simulink model "db4_14"  (R2018a)
settings: Solver=ode45  StartTime=0.0  StopTime=8  MaxStep=3e-5  RelTol=1e-3  AbsTol=1e-3
values from neighbouring files (symbols this model uses):
  Tc = str2num(get(findobj('Tag','variable6'),'String'))    [graficas_a.m]    (also in simulaciones.m = str2num(get(findobj('Tag','variable5'),'String')))
  Wref = str2num(get(findobj('Tag','variable5'),'String'))    [graficas_a.m]    (also in simulaciones.m)
libraries: simulink x2
settings Model: ExtModeTrigMode=oneshot  ExtModeArmWhenConnect=off  Creator=Lac User  LastModifiedBy=Matias
settings SolverCC: AutoScaleAbsTol=off
settings DataIOCC: SaveFormat=Array  SignalLoggingSaveFormat=ModelDataLogs  SaveOutput=off  SaveTime=off
settings OptimizationCC: BlockReduction=off  BooleanDataType=off  LifeSpan=inf
settings DebuggingCC: SaveWithParameterizedLinksMsg=none  UnderspecifiedInitializationDetection=Classic  MergeDetectMultiDrivingBlocksExec=none  SignalResolutionControl=TryResolveAllWithWarning  MultiTaskDSMMsg=warning  MultiTaskCondExecSysMsg=none  SFUnexpectedBacktrackingDiag=warning  SFNoUnconditionalDefaultTransitionDiag=warning  SFExecutionAtInitializationDiag=none
settings HardwareCC: ProdBitPerPointer=32  ProdBitPerSizeT=32  ProdBitPerPtrDiffT=32  ProdLargestAtomicFloat=None  ProdIntDivRoundTo=Undefined  ProdEndianess=Unspecified  ProdWordSize=32  ProdHWDeviceType=32-bit Generic  TargetUnknown=on
settings ModelReferenceCC: PropagateSignalLabelsOutOfModel=off
settings RTWCC: TemplateMakefile=grt_vc.tmf
settings CodeAppCC: StateflowObjectComments=on
settings GRTTargetCC: TargetLangStandard=C89/C90 (ANSI)  GeneratePreprocessorConditionals=Disable all  CombineOutputUpdateFcns=off  GRTInterface=on
settings ConfigComp: CovMetricSettings=dw  CovHtmlReporting=on  CovSaveCumulativeToWorkspaceVar=on  CovSaveSingleToWorkspaceVar=on  CovExternalEMLEnable=off

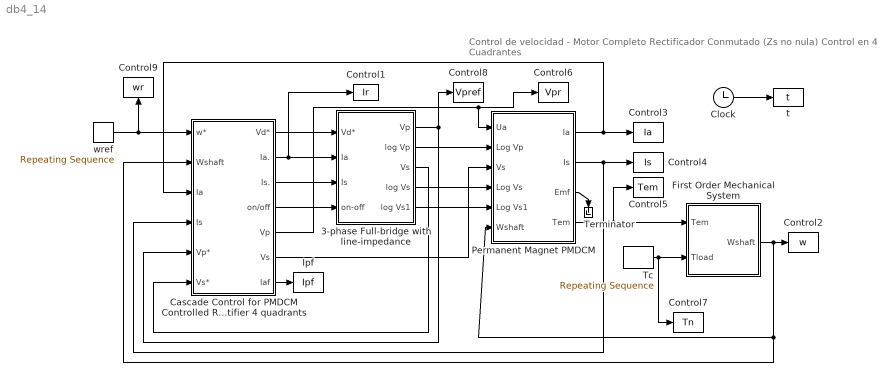
== system db4_14 ==
  note: Control de velocidad - Motor Completo
      | Rectificador Conmutado (Zs no nula) Control en 4 Cuadrantes
  3-phase Full-bridge with line-impedance : Subsystem  mask(3-phase Full-bridge with line-impedance){Vph=220, f=50, Rd=0.05, Ld=0.003, Rs=6e-05, Ls=2e-05}
      mask prompts: Vph "RMS Phase Voltage [V]:"; f "Frecuency [Hz]:"; Rd "Armature Resistance [Ohms]:"; Ld "Armature Inductance  [Hy]:"; Rs "Line Resistance [Ohms]:"; Ls "Line Inductance [Hy]:"
  "Cascade Control for PMDCM Controlled Rectifier 4 quadrants " : Subsystem  mask(Cascade Control (Speed and Current) for PMDCM Controlled Rectifier four quadrants){Kpn=283.88, TIn=0.3135, Kpi=0.08, TIi=0.027, Ktn=0.06, Tfn=0.008, Kti=1, Tfi=0.008, k=6.7851, Ian=319.6936}
      mask prompts: Kpn "Speed Proportional Gain:"; TIn "Speed Integral Gain:"; Kpi "Current Proportional Gain:"; TIi "Current Integral Gain:"; Ktn "Speed-sensor Proportional Gain:"; Tfn "Speed-sensor Integral Gain:"; Kti "Current-sensor Proportional Gain:"; Tfi "Current-sensor Integral Gain:"; k "Motor Constant:"; Ian "Rated Armature Current [Amp]:"
  Clock : Clock
  Control1 : ToWorkspace  VariableName=Ir
      settings: MaxDataPoints=300000
  Control2 : ToWorkspace  VariableName=w
      settings: MaxDataPoints=300000
  Control3 : ToWorkspace  VariableName=Ia
      settings: MaxDataPoints=300000
  Control4 : ToWorkspace  VariableName=Is
      settings: MaxDataPoints=300000
  Control5 : ToWorkspace  VariableName=Tem
      settings: MaxDataPoints=300000
  Control6 : ToWorkspace  VariableName=Vpr
      settings: MaxDataPoints=300000
  Control7 : ToWorkspace  VariableName=Tn
      settings: MaxDataPoints=300000
  Control8 : ToWorkspace  VariableName=Vpref
      settings: MaxDataPoints=300000
  Control9 : ToWorkspace  VariableName=wr
      settings: MaxDataPoints=300000
  First Order Mechanical System : Subsystem  mask(First Order Mechanical System){J=15, b=1.1, wor=0}
      mask prompts: J "Inertia [Kgm]:"; b "Friction Coeficient [Nm seg/rad]:"; wor "Speed Initial Condition [rad/sec]:"
      mask help:
      | This block solves the following differential equation:
      |
      | dW(t)/dt = - W(t)/J + (Tm -- bW(t) -- Load )/J
      | W(0)=W0
  Ipf : ToWorkspace  VariableName=Ipf
      settings: MaxDataPoints=300000
  Permanent Magnet PMDCM : Subsystem  mask(Permanent Magnet PMDCM){La=0.003, Ra=0.05, k=6.7851, ic=0, Ls=2e-05, Rs=6e-05}
      mask prompts: La "Armature Inductance  [Hy]:"; Ra "Armature Resistance [Ohms]:"; k "Motor Constant:"; ic "Armature Current Initial Condition [Amp]:"; Ls "Line Inductance [Hy]:"; Rs "Line Resistance [Ohms]:"
  Tc : simulink/Sources/Repeating Sequence  rep_seq_t=[0 7.5 7.9 8 9 9.1 10 13.5 14]  rep_seq_y="[0 0    0 -Tc -Tc -Tc -Tc -Tc 0]"
  Terminator : Terminator
  t : ToWorkspace  VariableName=t
      settings: MaxDataPoints=300000
  wref : simulink/Sources/Repeating Sequence  rep_seq_t="[0     1.5  2.5  3 4.5   5    6     8    9    10 11   12 15]"  rep_seq_y="[Wref Wref Wref  0  0    0   Wref   Wref Wref Wref  Wref   -Wref -Wref]"
  wires:
  wref/1 -> Control9/1, "Cascade Control for PMDCM Controlled Rectifier 4 quadrants "/1(w*)
  "Cascade Control for PMDCM Controlled Rectifier 4 quadrants "/7(Iaf) -> Ipf/1
  First Order Mechanical System/1(Wshaft) -> Permanent Magnet PMDCM/6(Wshaft), "Cascade Control for PMDCM Controlled Rectifier 4 quadrants "/2(Wshaft), Control2/1
  "Cascade Control for PMDCM Controlled Rectifier 4 quadrants "/1(Vd*) -> 3-phase Full-bridge with line-impedance/1(Vd*)
  "Cascade Control for PMDCM Controlled Rectifier 4 quadrants "/4(on/off) -> 3-phase Full-bridge with line-impedance/4(on-off)
  "Cascade Control for PMDCM Controlled Rectifier 4 quadrants "/3(Is.) -> 3-phase Full-bridge with line-impedance/3(Is)
  3-phase Full-bridge with line-impedance/3(Vs) -> "Cascade Control for PMDCM Controlled Rectifier 4 quadrants "/6(Vs*)
  "Cascade Control for PMDCM Controlled Rectifier 4 quadrants "/6(Vs) -> Permanent Magnet PMDCM/3(Vs)
  3-phase Full-bridge with line-impedance/5(log Vs1) -> Permanent Magnet PMDCM/5(Log Vs1)
  3-phase Full-bridge with line-impedance/4(log Vs) -> Permanent Magnet PMDCM/4(Log Vs)
  "Cascade Control for PMDCM Controlled Rectifier 4 quadrants "/5(Vp) -> Permanent Magnet PMDCM/1(Ua), Control6/1
  3-phase Full-bridge with line-impedance/2(log Vp) -> Permanent Magnet PMDCM/2(Log Vp)
  "Cascade Control for PMDCM Controlled Rectifier 4 quadrants "/2(Ia.) -> 3-phase Full-bridge with line-impedance/2(Ia), Control1/1
  3-phase Full-bridge with line-impedance/1(Vp) -> "Cascade Control for PMDCM Controlled Rectifier 4 quadrants "/5(Vp*), Control8/1
  Permanent Magnet PMDCM/3(Emf) -> Terminator/1
  Permanent Magnet PMDCM/2(Is) -> Control4/1, "Cascade Control for PMDCM Controlled Rectifier 4 quadrants "/4(Is)
  Permanent Magnet PMDCM/1(Ia) -> Control3/1, "Cascade Control for PMDCM Controlled Rectifier 4 quadrants "/3(Ia)
  Permanent Magnet PMDCM/4(Tem) -> First Order Mechanical System/1(Tem), Control5/1
  Tc/1 -> First Order Mechanical System/2(Tload), Control7/1
  Clock/1 -> t/1

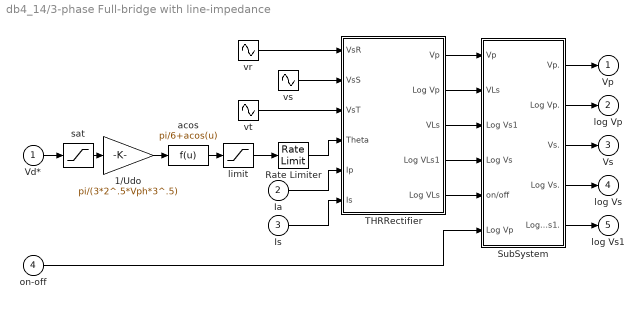
== system db4_14/3-phase Full-bridge with line-impedance ==
  Vd* : Inport
  Ia : Inport  Port=2
  Is : Inport  Port=3
  on-off : Inport  Port=4
  1/Udo : Gain  Gain=pi/(3*2^.5*Vph*3^.5)  SaturateOnIntegerOverflow=on  OutDataTypeStr=Inherit: Same as input  ParamDataTypeStr=Inherit: Same as input
  Rate Limiter : RateLimiter  RisingSlewLimit=8000  FallingSlewLimit=-8000
  SubSystem : Subsystem
  THRRectifier : Subsystem
      mask Display:
      | plot([0.3 0.7 0.5 0.3],[0.4 0.4 0.6 0.4])
      | plot([0.3 0.7 ],[0.6 0.6])
      | plot([0.5 0.5 ],[0.6 0.7])
      | plot([0.5 0.5 ],[0.3 0.4])
      | plot([0.35 0.5],[0.7 0.6])
      | plot([0.25 0.35 ],[0.7 0.7])
  acos : Fcn  Expr=pi/6+acos(u)
  limit : Saturate  UpperLimit=pi*6.999/6  LowerLimit=pi/5.998
  sat : Saturate  UpperLimit=(3*2^.5*3^.5*Vph)/pi  LowerLimit=-(3*2^.5*3^.5*Vph)/pi
  vr : Sin  Amplitude=Vph*(2^.5)  Frequency=2*f*pi  SampleTime=0
  vs : Sin  Amplitude=Vph*(2^.5)  Frequency=2*pi*f  Phase=-(2/3)*pi  SampleTime=0
  vt : Sin  Amplitude=Vph*(2^.5)  Frequency=2*pi*f  Phase=-(4/3)*pi  SampleTime=0
  Vp : Outport
  log Vp : Outport  Port=2
  Vs : Outport  Port=3
  log Vs : Outport  Port=4
  log Vs1 : Outport  Port=5
  wires:
  1/Udo/1 -> acos/1
  acos/1 -> limit/1
  vt/1 -> THRRectifier/3(VsT)
  vs/1 -> THRRectifier/2(VsS)
  vr/1 -> THRRectifier/1(VsR)
  Vd*/1 -> sat/1
  Ia/1 -> THRRectifier/5(Ip)
  Is/1 -> THRRectifier/6(Is)
  sat/1 -> 1/Udo/1
  limit/1 -> Rate Limiter/1
  THRRectifier/1(Vp) -> SubSystem/1(Vp)
  THRRectifier/2(Log Vp) -> SubSystem/2(VLs)
  THRRectifier/3(VLs) -> SubSystem/3(Log Vs1)
  THRRectifier/4(Log VLs1) -> SubSystem/4(Log Vs)
  THRRectifier/5(Log VLs) -> SubSystem/5(on/off)
  on-off/1 -> SubSystem/6(Log Vp)
  SubSystem/2(Log Vp.) -> log Vp/1
  SubSystem/3(Vs.) -> Vs/1
  SubSystem/4(Log Vs.) -> log Vs/1
  SubSystem/5(Log Vs1.) -> log Vs1/1
  SubSystem/1(Vp.) -> Vp/1
  Rate Limiter/1 -> THRRectifier/4(Theta)

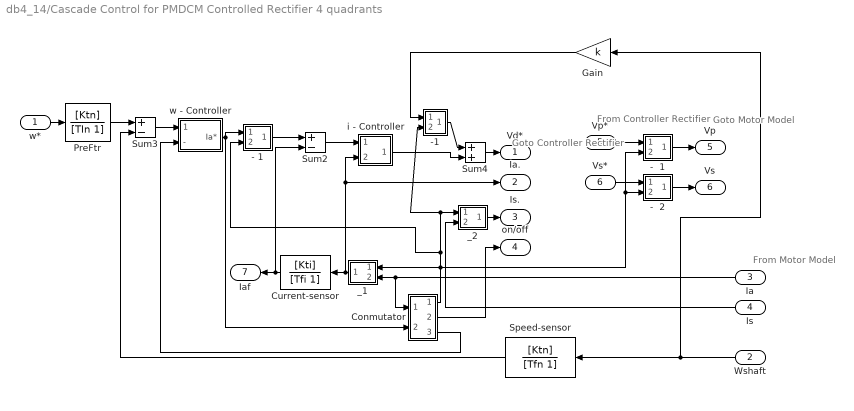
== system db4_14/Cascade Control for PMDCM Controlled Rectifier 4 quadrants  ==
  note: From Controller
      | Rectifier
  note: Goto Motor
      | Model
  note: Goto Controller
      | Rectifier
  note: From Motor
      | Model
  w* : Inport
  Wshaft : Inport  Port=2
  Ia : Inport  Port=3
  Is : Inport  Port=4
  Vp* : Inport  Port=5
  Vs* : Inport  Port=6
  -  1 : Subsystem
      mask Display: disp('-1')
  -  2 : Subsystem
      mask Display: disp('-1')
  - 1 : Subsystem
      mask Display: disp('-1')
  -1 : Subsystem
      mask Display: disp('-1')
  Conmutator : Subsystem
  Current-sensor : TransferFcn  Numerator=[Kti]  Denominator=[Tfi 1]
  Gain : Gain  Gain=k  SaturateOnIntegerOverflow=on  OutDataTypeStr=Inherit: Same as input  ParamDataTypeStr=Inherit: Same as input
  PreFtr : TransferFcn  Numerator=[Ktn]  Denominator=[TIn 1]
  Speed-sensor : TransferFcn  Numerator=[Ktn]  Denominator=[Tfn 1]
  Sum2 : Sum  Inputs=+-  SaturateOnIntegerOverflow=on  InputSameDT=on  OutDataTypeStr=Inherit: Same as first input
  Sum3 : Sum  Inputs=+-  SaturateOnIntegerOverflow=on  InputSameDT=on  OutDataTypeStr=Inherit: Same as first input
  Sum4 : Sum  SaturateOnIntegerOverflow=on  InputSameDT=on  OutDataTypeStr=Inherit: Same as first input
  _1 : Subsystem
      mask Display: disp('-1')
  _2 : Subsystem
      mask Display: disp('-1')
  i - Controller : Subsystem
      mask Display: plot([0 .01  5],[0 2 4])
  w - Controller : Subsystem
      mask Display:
      | plot([0.1 .1  0.6],[0.1 .5 .9])
      | plot([0.85 0.95],[0.65 0.65])
      | plot([0.8 0.85],[0.75 0.65])
      | plot([0.95 1],[0.65 0.75])
      | plot([0.85 0.95],[0.35 0.35])
      | plot([0.80 0.85],[0.25 0.35])
      | plot([0.95 1],[0.35 0.25])
      | plot([0.7 1], [0.5 .5])
      | plot([0 0], [0 1])
      | plot([0 0.7], [1 1])
      | plot([0.7 0.7], [0 1])
      | plot([0 0.7], [0 0])
  Vd* : Outport
  Ia. : Outport  Port=2
  Is. : Outport  Port=3
  on/off : Outport  Port=4
  Vp : Outport  Port=5
  Vs : Outport  Port=6
  Iaf : Outport  Port=7
  wires:
  Speed-sensor/1 -> Sum3/2
  PreFtr/1 -> Sum3/1
  _1/1(out_1) -> Current-sensor/1, i - Controller/2(Ia), Ia./1
  Sum2/1 -> i - Controller/1(Iaref - Iaf)
  Sum3/1 -> w - Controller/1(w - Iref)
  Conmutator/3(Ir = 0) -> w - Controller/2(-)
  w*/1 -> PreFtr/1
  - 1/1(out_1) -> Sum2/1
  Conmutator/2(Vp*1) -> on/off/1
  w - Controller/1(Ia*) -> - 1/1(in_1), Conmutator/2(Iaref)
  Conmutator/1(Vp*) -> - 1/2(in_2), _2/1(in_2), -1/2(in_2), -  2/2(in_2), -  1/2(in_2), _1/1(in_2)
  Vp*/1 -> -  1/1(in_1)
  Vs*/1 -> -  2/1(in_1)
  -  1/1(out_1) -> Vp/1
  -  2/1(out_1) -> Vs/1
  _2/1(out_1) -> Is./1
  Is/1 -> _2/2(in_1)
  Gain/1 -> -1/1(in_1)
  -1/1(out_1) -> Sum4/1
  i - Controller/1(Vp*) -> Sum4/2
  Sum4/1 -> Vd*/1
  Ia/1 -> _1/2(in_1), Conmutator/1(Ia)
  Wshaft/1 -> Speed-sensor/1, Gain/1
  Current-sensor/1 -> Sum2/2, Iaf/1

== system db4_14/First Order Mechanical System ==
  Tem : Inport
  Tload : Inport  Port=2
  Gain : Gain  Gain=1/J  SaturateOnIntegerOverflow=on  OutDataTypeStr=Inherit: Same as input  ParamDataTypeStr=Inherit: Same as input
  Gain1 : Gain  Gain=b  SaturateOnIntegerOverflow=on  OutDataTypeStr=Inherit: Same as input  ParamDataTypeStr=Inherit: Same as input
  Integrator : Integrator  InitialCondition=wor
  Sum : Sum  Inputs=+--  SaturateOnIntegerOverflow=on  InputSameDT=on  OutDataTypeStr=Inherit: Same as first input
  Wshaft : Outport
  wires:
  Integrator/1 -> Wshaft/1, Gain1/1
  Gain1/1 -> Sum/3
  Gain/1 -> Integrator/1
  Sum/1 -> Gain/1
  Tem/1 -> Sum/1
  Tload/1 -> Sum/2

== system db4_14/Permanent Magnet PMDCM ==
  Ua : Inport
  Log Vp : Inport  Port=2
  Vs : Inport  Port=3
  Log Vs : Inport  Port=4
  Log Vs1 : Inport  Port=5
  Wshaft : Inport  Port=6
  Converter with Zs 2 & 4 Quadrants : Subsystem
  Gain6 : Gain  Gain=k  SaturateOnIntegerOverflow=on  OutDataTypeStr=Inherit: Same as input  ParamDataTypeStr=Inherit: Same as input
  k : Gain  Gain=k  SaturateOnIntegerOverflow=on  OutDataTypeStr=Inherit: Same as input  ParamDataTypeStr=Inherit: Same as input
  Ia : Outport
  Is : Outport  Port=2
  Emf : Outport  Port=3
  Tem : Outport  Port=4
  wires:
  k/1 -> Converter with Zs 2 & 4 Quadrants/1(e), Emf/1
  Ua/1 -> Converter with Zs 2 & 4 Quadrants/2(Vp)
  Log Vp/1 -> Converter with Zs 2 & 4 Quadrants/3(LogVp)
  Vs/1 -> Converter with Zs 2 & 4 Quadrants/4(Vs)
  Log Vs/1 -> Converter with Zs 2 & 4 Quadrants/5(LogVs)
  Log Vs1/1 -> Converter with Zs 2 & 4 Quadrants/6(LogVs1)
  Wshaft/1 -> k/1
  Converter with Zs 2 & 4 Quadrants/2(Is) -> Is/1
  Gain6/1 -> Tem/1
  Converter with Zs 2 & 4 Quadrants/1(Ip) -> Ia/1, Gain6/1

== system db4_14/3-phase Full-bridge with line-impedance/SubSystem ==
  Vp : Inport
  VLs : Inport  Port=2
  Log Vs1 : Inport  Port=3
  Log Vs : Inport  Port=4
  on/off : Inport  Port=5
  Log Vp : Inport  Port=6
  Product{1..5} (5 alike) : Product  SaturateOnIntegerOverflow=on  RndMeth=Zero  InputSameDT=on  OutDataTypeStr=Inherit: Same as first input
  Vp. : Outport
  Log Vp. : Outport  Port=2
  Vs. : Outport  Port=3
  Log Vs. : Outport  Port=4
  Log Vs1. : Outport  Port=5
  wires:
  VLs/1 -> Product2/2
  Log Vp/1 -> Product1/2, Product2/1, Product5/1, Product4/1, Product3/1
  Product2/1 -> Log Vp./1
  Product1/1 -> Vp./1
  Vp/1 -> Product1/1
  Log Vs1/1 -> Product3/2
  Log Vs/1 -> Product4/2
  on/off/1 -> Product5/2
  Product5/1 -> Log Vs1./1
  Product4/1 -> Log Vs./1
  Product3/1 -> Vs./1

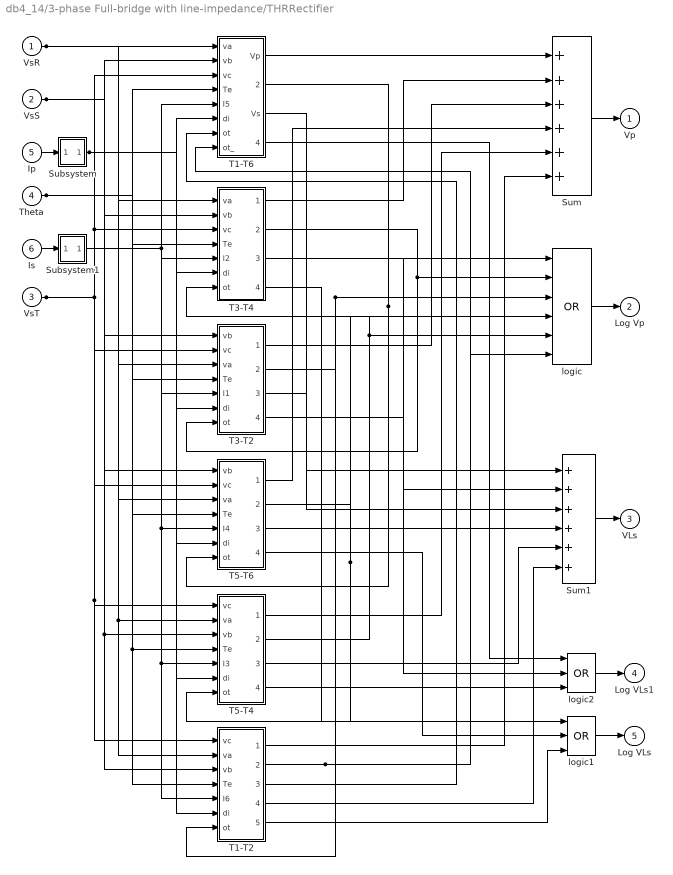
== system db4_14/3-phase Full-bridge with line-impedance/THRRectifier ==
  VsR : Inport
  VsS : Inport  Port=2
  VsT : Inport  Port=3
  Theta : Inport  Port=4
  Ip : Inport  Port=5
  Is : Inport  Port=6
  Subsystem : Subsystem
  Subsystem1 : Subsystem
  Sum : Sum  Inputs=++++++  SaturateOnIntegerOverflow=on  InputSameDT=on  OutDataTypeStr=Inherit: Same as first input
  Sum1 : Sum  Inputs=++++++  SaturateOnIntegerOverflow=on  InputSameDT=on  OutDataTypeStr=Inherit: Same as first input
  T1-T2 : Subsystem
  T1-T6 : Subsystem
  T3-T2 : Subsystem
  T3-T4 : Subsystem
  T5-T4 : Subsystem
  T5-T6 : Subsystem
  logic : Logic  Operator=OR  Inputs=6
  logic1 : Logic  Operator=OR  Inputs=3
  logic2 : Logic  Operator=OR  Inputs=3
  Vp : Outport
  Log Vp : Outport  Port=2
  VLs : Outport  Port=3
  Log VLs1 : Outport  Port=4
  Log VLs : Outport  Port=5
  wires:
  logic2/1 -> Log VLs1/1
  logic1/1 -> Log VLs/1
  Subsystem1/1(out_1) -> T1-T6/5(I5), T1-T2/5(I6), T5-T4/5(I3), T5-T6/5(I4), T3-T4/5(I2), T3-T2/5(I1)
  Subsystem/1(out_1) -> T5-T4/6(di), T5-T6/6(di), T3-T2/6(di), T3-T4/6(di), T1-T6/6(di), T1-T2/6(di)
  Theta/1 -> T1-T2/4(Te), T5-T4/4(Te), T5-T6/4(Te), T3-T2/4(Te), T3-T4/4(Te), T1-T6/4(Te)
  T1-T2/2(out_1) -> T1-T6/8(ot_), logic/6
  logic/1 -> Log Vp/1
  Sum/1 -> Vp/1
  Ip/1 -> Subsystem/1(in_1)
  Sum1/1 -> VLs/1
  T1-T6/2(Log Vp) -> T5-T6/7(ot), logic/1
  T1-T6/1(Vp) -> Sum/1
  T1-T6/3(Vs) -> Sum1/1
  T1-T6/4(Log Vs) -> logic2/1
  T3-T4/1(out_2) -> Sum/2
  VsR/1 -> T1-T6/1(va), T3-T4/1(va), T3-T2/3(va), T5-T6/3(va), T5-T4/2(va), T1-T2/2(va)
  VsS/1 -> T1-T6/2(vb), T3-T4/2(vb), T3-T2/1(vb), T5-T6/1(vb), T5-T4/3(vb), T1-T2/3(vb)
  T3-T4/2(out_1) -> T3-T2/7(ot), logic/2
  T3-T4/3(out_3) -> Sum1/2
  T3-T4/4(out_4) -> logic1/1
  T3-T2/1(out_2) -> Sum/3
  T3-T2/2(out_1) -> logic/3, T1-T2/7(ot)
  T3-T2/3(out_3) -> Sum1/3
  T3-T2/4(out_4) -> logic2/2
  VsT/1 -> T3-T2/2(vc), T1-T6/3(vc), T3-T4/3(vc), T5-T6/2(vc), T5-T4/1(vc), T1-T2/1(vc)
  T5-T6/2(out_1) -> T5-T4/7(ot), logic/4
  T5-T6/3(out_3) -> Sum1/4
  T5-T6/4(out_4) -> logic1/2
  T5-T6/1(out_2) -> Sum/4
  T5-T4/2(out_1) -> T3-T4/7(ot), logic/5
  T5-T4/1(out_2) -> Sum/5
  T5-T4/3(out_3) -> Sum1/5
  T5-T4/4(out_4) -> logic2/3
  T1-T2/3(out_3) -> T1-T6/7(ot)
  T1-T2/4("out_4 ") -> Sum1/6
  T1-T2/5(out_5) -> logic1/3
  T1-T2/1(out_2) -> Sum/6
  Is/1 -> Subsystem1/1(in_1)

== system db4_14/Cascade Control for PMDCM Controlled Rectifier 4 quadrants /-  1 ==
  in_1 : Inport
  in_2 : Inport  Port=2
  Gain1 : Gain  Gain=-1  SaturateOnIntegerOverflow=on  OutDataTypeStr=Inherit: Same as input  ParamDataTypeStr=Inherit: Same as input
  Switch1 : Switch  Threshold=.5  SaturateOnIntegerOverflow=on  InputSameDT=on
  out_1 : Outport
  wires:
  in_1/1 -> Gain1/1, Switch1/1
  Gain1/1 -> Switch1/3
  Switch1/1 -> out_1/1
  in_2/1 -> Switch1/2

== system db4_14/Cascade Control for PMDCM Controlled Rectifier 4 quadrants /-  2 ==
  in_1 : Inport
  in_2 : Inport  Port=2
  Gain1 : Gain  Gain=-1  SaturateOnIntegerOverflow=on  OutDataTypeStr=Inherit: Same as input  ParamDataTypeStr=Inherit: Same as input
  Switch1 : Switch  Threshold=.5  SaturateOnIntegerOverflow=on  InputSameDT=on
  out_1 : Outport
  wires:
  in_2/1 -> Switch1/2
  Switch1/1 -> out_1/1
  Gain1/1 -> Switch1/3
  in_1/1 -> Gain1/1, Switch1/1

== system db4_14/Cascade Control for PMDCM Controlled Rectifier 4 quadrants /- 1 ==
  in_1 : Inport
  in_2 : Inport  Port=2
  Gain1 : Gain  Gain=-1  SaturateOnIntegerOverflow=on  OutDataTypeStr=Inherit: Same as input  ParamDataTypeStr=Inherit: Same as input
  Switch1 : Switch  Threshold=.5  SaturateOnIntegerOverflow=on  InputSameDT=on
  out_1 : Outport
  wires:
  in_2/1 -> Switch1/2
  Switch1/1 -> out_1/1
  Gain1/1 -> Switch1/3
  in_1/1 -> Gain1/1, Switch1/1

== system db4_14/Cascade Control for PMDCM Controlled Rectifier 4 quadrants /-1 ==
  in_1 : Inport
  in_2 : Inport  Port=2
  Gain1 : Gain  Gain=-1  SaturateOnIntegerOverflow=on  OutDataTypeStr=Inherit: Same as input  ParamDataTypeStr=Inherit: Same as input
  Switch1 : Switch  Threshold=.5  SaturateOnIntegerOverflow=on  InputSameDT=on
  out_1 : Outport
  wires:
  in_2/1 -> Switch1/2
  Switch1/1 -> out_1/1
  Gain1/1 -> Switch1/3
  in_1/1 -> Gain1/1, Switch1/1

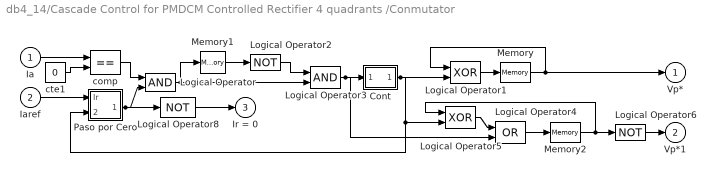
== system db4_14/Cascade Control for PMDCM Controlled Rectifier 4 quadrants /Conmutator ==
  Ia : Inport
  Iaref : Inport  Port=2
  Cont : Subsystem
  Logical Operator : Logic
  Logical Operator1 : Logic  Operator=XOR
  Logical Operator2 : Logic  Operator=NOT  Inputs=1
  Logical Operator3 : Logic
  Logical Operator4 : Logic  Operator=OR
  Logical Operator5 : Logic  Operator=XOR
  Logical Operator6 : Logic  Operator=NOT  Inputs=1
  Logical Operator8 : Logic  Operator=NOT  Inputs=1
  Memory : Memory
  Memory1 : Memory  InitialCondition=1
  Memory2 : Memory  InitialCondition=1
  Paso por Cero : Subsystem
  comp : RelationalOperator  Operator===  RndMeth=Nearest  InputSameDT=on
  cte1 : Constant  Value=0
  Vp* : Outport
  Vp*1 : Outport  Port=2
  Ir = 0 : Outport  Port=3
  wires:
  Logical Operator8/1 -> Ir = 0/1
  Paso por Cero/1(Ir = 0) -> Logical Operator8/1, Logical Operator/2
  Memory/1 -> Vp*/1, Logical Operator1/1
  Memory2/1 -> Logical Operator6/1, Logical Operator5/1
  Logical Operator4/1 -> Memory2/1
  Logical Operator6/1 -> Vp*1/1
  Logical Operator3/1 -> Logical Operator4/2, Cont/1(in_2)
  Cont/1(out_1) -> Paso por Cero/2(Cont), Logical Operator5/2, Logical Operator1/2
  Logical Operator5/1 -> Logical Operator4/1
  comp/1 -> Logical Operator/1
  Logical Operator2/1 -> Logical Operator3/1
  Logical Operator/1 -> Logical Operator3/2, Memory1/1
  Memory1/1 -> Logical Operator2/1
  Logical Operator1/1 -> Memory/1
  Iaref/1 -> Paso por Cero/1(Ir)
  Ia/1 -> comp/1
  cte1/1 -> comp/2

== system db4_14/Cascade Control for PMDCM Controlled Rectifier 4 quadrants /_1 ==
  in_2 : Inport
  in_1 : Inport  Port=2
  Gain1 : Gain  Gain=-1  SaturateOnIntegerOverflow=on  OutDataTypeStr=Inherit: Same as input  ParamDataTypeStr=Inherit: Same as input
  Switch1 : Switch  Threshold=.5  SaturateOnIntegerOverflow=on  InputSameDT=on
  out_1 : Outport
  wires:
  in_2/1 -> Switch1/2
  Switch1/1 -> out_1/1
  Gain1/1 -> Switch1/3
  in_1/1 -> Gain1/1, Switch1/1

== system db4_14/Cascade Control for PMDCM Controlled Rectifier 4 quadrants /_2 ==
  in_2 : Inport
  in_1 : Inport  Port=2
  Gain1 : Gain  Gain=-1  SaturateOnIntegerOverflow=on  OutDataTypeStr=Inherit: Same as input  ParamDataTypeStr=Inherit: Same as input
  Switch1 : Switch  Threshold=.5  SaturateOnIntegerOverflow=on  InputSameDT=on
  out_1 : Outport
  wires:
  in_1/1 -> Gain1/1, Switch1/1
  Gain1/1 -> Switch1/3
  Switch1/1 -> out_1/1
  in_2/1 -> Switch1/2

== system db4_14/Cascade Control for PMDCM Controlled Rectifier 4 quadrants /i - Controller ==
  Iaref - Iaf : Inport
  Ia : Inport  Port=2
  I -ctrl : Subsystem
  comp : RelationalOperator  Operator=>  RndMeth=Nearest  InputSameDT=on
  cte1 : Constant  Value=0
  sat : Saturate  UpperLimit=514.598  LowerLimit=-514.598
  Vp* : Outport
  wires:
  Iaref - Iaf/1 -> I -ctrl/2(in_1)
  cte1/1 -> comp/2
  sat/1 -> Vp*/1
  I -ctrl/1(out_1) -> sat/1
  comp/1 -> I -ctrl/1(in_2)
  Ia/1 -> comp/1

== system db4_14/Cascade Control for PMDCM Controlled Rectifier 4 quadrants /w - Controller ==
  w - Iref : Inport
  - : Inport  Port=2
  Gain : Gain  Gain=Kpn/TIn  SaturateOnIntegerOverflow=on  OutDataTypeStr=Inherit: Same as input  ParamDataTypeStr=Inherit: Same as input
  Gain2 : Gain  Gain=Kpn  SaturateOnIntegerOverflow=on  OutDataTypeStr=Inherit: Same as input  ParamDataTypeStr=Inherit: Same as input
  Limited Integrator : Integrator  LimitOutput=on  UpperSaturationLimit=2*Ian  LowerSaturationLimit=-2*Ian
  Sum1 : Sum  SaturateOnIntegerOverflow=on  InputSameDT=on  OutDataTypeStr=Inherit: Same as first input
  mantiene salida = 0 : Product  SaturateOnIntegerOverflow=on  RndMeth=Zero  InputSameDT=on  OutDataTypeStr=Inherit: Same as first input
  sat : Saturate  UpperLimit=2*Ian  LowerLimit=-2*Ian
  Ia* : Outport
  wires:
  Gain2/1 -> Sum1/2
  Limited Integrator/1 -> Sum1/1
  -/1 -> mantiene salida = 0/1
  mantiene salida = 0/1 -> Ia*/1
  sat/1 -> mantiene salida = 0/2
  w - Iref/1 -> Gain2/1, Gain/1
  Sum1/1 -> sat/1
  Gain/1 -> Limited Integrator/1

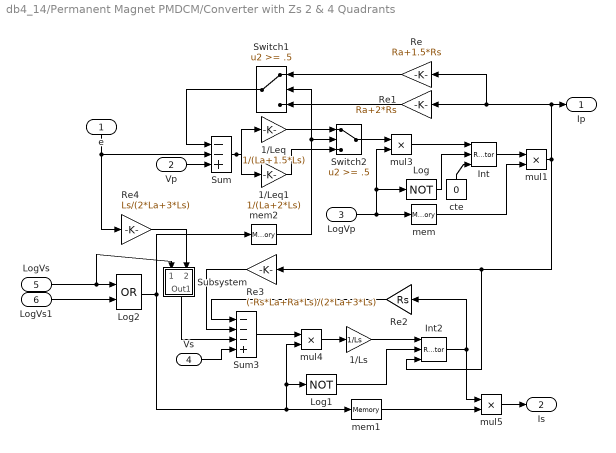
== system db4_14/Permanent Magnet PMDCM/Converter with Zs 2 & 4 Quadrants ==
  e : Inport
  Vp : Inport  Port=2
  LogVp : Inport  Port=3
  Vs : Inport  Port=4
  LogVs : Inport  Port=5
  LogVs1 : Inport  Port=6
  "1/Leq " : Gain  Gain=1/(La+1.5*Ls)  SaturateOnIntegerOverflow=on  OutDataTypeStr=Inherit: Same as input  ParamDataTypeStr=Inherit: Same as input
  1/Leq1 : Gain  Gain=1/(La+2*Ls)  SaturateOnIntegerOverflow=on  OutDataTypeStr=Inherit: Same as input  ParamDataTypeStr=Inherit: Same as input
  1/Ls : Gain  Gain=1/Ls  SaturateOnIntegerOverflow=on  OutDataTypeStr=Inherit: Same as input  ParamDataTypeStr=Inherit: Same as input
  Int : ResetIntegrator
  Int2 : ResetIntegrator
  Log : Logic  Operator=NOT  Inputs=1
  Log1 : Logic  Operator=NOT  Inputs=1
  Log2 : Logic  Operator=OR
  Re : Gain  Gain=Ra+1.5*Rs  SaturateOnIntegerOverflow=on  OutDataTypeStr=Inherit: Same as input  ParamDataTypeStr=Inherit: Same as input
  Re1 : Gain  Gain=Ra+2*Rs  SaturateOnIntegerOverflow=on  OutDataTypeStr=Inherit: Same as input  ParamDataTypeStr=Inherit: Same as input
  Re2 : Gain  Gain=Rs  SaturateOnIntegerOverflow=on  OutDataTypeStr=Inherit: Same as input  ParamDataTypeStr=Inherit: Same as input
  Re3 : Gain  Gain=(-Rs*La+Ra*Ls)/(2*La+3*Ls)  SaturateOnIntegerOverflow=on  OutDataTypeStr=Inherit: Same as input  ParamDataTypeStr=Inherit: Same as input
  Re4 : Gain  Gain=Ls/(2*La+3*Ls)  SaturateOnIntegerOverflow=on  OutDataTypeStr=Inherit: Same as input  ParamDataTypeStr=Inherit: Same as input
  Subsystem : Subsystem
      mask Display: disp('-1')
  Sum : Sum  Inputs=--+  SaturateOnIntegerOverflow=on  InputSameDT=on  OutDataTypeStr=Inherit: Same as first input
  Sum3 : Sum  Inputs=---+  SaturateOnIntegerOverflow=on  InputSameDT=on  OutDataTypeStr=Inherit: Same as first input
  Switch1 : Switch  Threshold=.5  SaturateOnIntegerOverflow=on  InputSameDT=on
  Switch2 : Switch  Threshold=.5  SaturateOnIntegerOverflow=on  InputSameDT=on
  cte : Constant  Value=0
  mem : Memory
  mem1 : Memory
  mem2 : Memory
  mul{1,3..5} (4 alike) : Product  SaturateOnIntegerOverflow=on  RndMeth=Zero  InputSameDT=on  OutDataTypeStr=Inherit: Same as first input
  Ip : Outport
  Is : Outport  Port=2
  wires:
  mem/1 -> mul1/2
  Int/1 -> mul1/1
  mul3/1 -> Int/1
  Log/1 -> Int/2
  cte/1 -> Int/3
  mul1/1 -> Re3/1, Int2/3, Ip/1, Re1/1, Re/1
  LogVp/1 -> mem/1, mul3/2, Log/1
  Switch2/1 -> mul3/1
  1/Leq1/1 -> Switch2/3
  "1/Leq "/1 -> Switch2/1
  Re/1 -> Switch1/1
  Re1/1 -> Switch1/3
  Vp/1 -> Sum/3
  mem2/1 -> Switch1/2, Switch2/2
  Sum/1 -> 1/Leq1/1, "1/Leq "/1
  Re3/1 -> Sum3/2
  Switch1/1 -> Sum/1
  LogVs/1 -> Subsystem/1(In1), Log2/1
  Vs/1 -> Sum3/4
  mul5/1 -> Is/1
  Re4/1 -> Subsystem/2(In2)
  Log2/1 -> mem2/1, mul4/2, Log1/1, mem1/1
  1/Ls/1 -> Int2/1
  mul4/1 -> 1/Ls/1
  Log1/1 -> Int2/2
  Re2/1 -> Sum3/1
  Sum3/1 -> mul4/1
  mem1/1 -> mul5/2
  Int2/1 -> Re2/1, mul5/1
  e/1 -> Sum/2, Re4/1
  Subsystem/1(Out1) -> Sum3/3
  LogVs1/1 -> Log2/2

== system db4_14/3-phase Full-bridge with line-impedance/THRRectifier/Subsystem ==
  in_1 : Inport
  comp : RelationalOperator  Operator=>  RndMeth=Nearest  InputSameDT=on
  cte : Constant  Value=0
  out_1 : Outport
  wires:
  cte/1 -> comp/2
  in_1/1 -> comp/1
  comp/1 -> out_1/1

== system db4_14/3-phase Full-bridge with line-impedance/THRRectifier/Subsystem1 ==
  in_1 : Inport
  Vdset : Step  Time=0  Before=1  SampleTime=0
  comp : RelationalOperator  Operator=>  RndMeth=Nearest  InputSameDT=on
  cte : Constant  Value=0
  mul : Product  SaturateOnIntegerOverflow=on  RndMeth=Zero  InputSameDT=on  OutDataTypeStr=Inherit: Same as first input
  out_1 : Outport
  wires:
  Vdset/1 -> mul/2
  mul/1 -> out_1/1
  comp/1 -> mul/1
  cte/1 -> comp/2
  in_1/1 -> comp/1

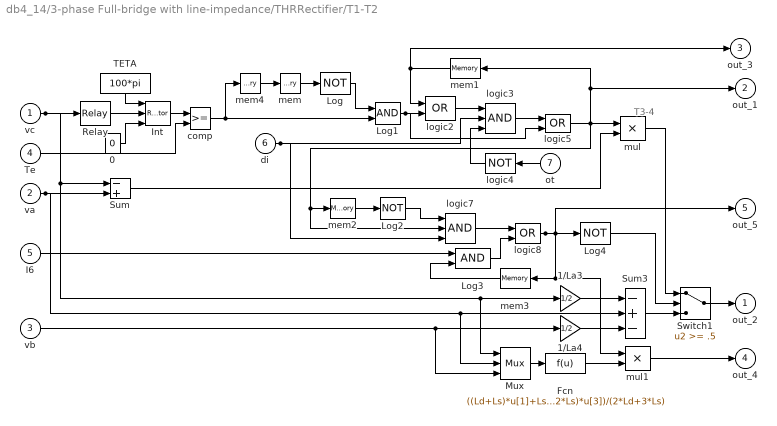
== system db4_14/3-phase Full-bridge with line-impedance/THRRectifier/T1-T2 ==
  note: T3-4
  vc : Inport
  va : Inport  Port=2
  vb : Inport  Port=3
  Te : Inport  Port=4
  I6 : Inport  Port=5
  di : Inport  Port=6
  ot : Inport  Port=7
  0 : Constant  Value=0
  1/La3 : Gain  Gain=1/2  SaturateOnIntegerOverflow=on  OutDataTypeStr=Inherit: Same as input  ParamDataTypeStr=Inherit: Same as input
  1/La4 : Gain  Gain=1/2  SaturateOnIntegerOverflow=on  OutDataTypeStr=Inherit: Same as input  ParamDataTypeStr=Inherit: Same as input
  Fcn : Fcn  Expr=((Ld+Ls)*u[1]+Ls*u[2]-(Ld+2*Ls)*u[3])/(2*Ld+3*Ls)
  Int : ResetIntegrator
  Log : Logic  Operator=NOT  Inputs=1
  Log1 : Logic
  Log2 : Logic  Operator=NOT  Inputs=1
  Log3 : Logic
  Log4 : Logic  Operator=NOT  Inputs=1
  Mux : Mux  Inputs=3
  Relay : Relay  OnSwitchValue=(2^.5)*Vph*sin(pi/6)  OffSwitchValue=0
  Sum : Sum  Inputs=-+  SaturateOnIntegerOverflow=on  InputSameDT=on  OutDataTypeStr=Inherit: Same as first input
  Sum3 : Sum  Inputs=-+-  SaturateOnIntegerOverflow=on  InputSameDT=on  OutDataTypeStr=Inherit: Same as first input
  Switch1 : Switch  Threshold=.5  SaturateOnIntegerOverflow=on  InputSameDT=on
  TETA : Constant  Value=100*pi
  comp : RelationalOperator  RndMeth=Nearest  InputSameDT=on
  logic2 : Logic  Operator=OR
  logic3 : Logic  Inputs=3
  logic4 : Logic  Operator=NOT  Inputs=1
  logic5 : Logic  Operator=OR
  logic7 : Logic  Inputs=3
  logic8 : Logic  Operator=OR
  mem{,1..4} (5 alike) : Memory
  mul : Product  SaturateOnIntegerOverflow=on  RndMeth=Zero  InputSameDT=on  OutDataTypeStr=Inherit: Same as first input
  mul1 : Product  SaturateOnIntegerOverflow=on  RndMeth=Zero  InputSameDT=on  OutDataTypeStr=Inherit: Same as first input
  out_2 : Outport
  out_1 : Outport  Port=2
  out_3 : Outport  Port=3
  "out_4 " : Outport  Port=4
  out_5 : Outport  Port=5
  wires:
  comp/1 -> Log1/2, mem4/1
  mem4/1 -> mem/1
  mem/1 -> Log/1
  logic4/1 -> logic3/3
  0/1 -> Int/3
  logic2/1 -> logic3/1
  TETA/1 -> Int/1
  Int/1 -> comp/1
  Te/1 -> comp/2
  ot/1 -> logic4/1
  Relay/1 -> Int/2
  logic3/1 -> logic5/1
  Log1/1 -> logic2/2, logic5/2
  logic5/1 -> mul/1, mem2/1, logic7/2, mem1/1, out_1/1
  mem2/1 -> Log2/1
  Log/1 -> Log1/1
  Log3/1 -> logic8/2
  logic7/1 -> logic8/1
  di/1 -> logic3/2, logic7/3
  Log2/1 -> logic7/1
  1/La4/1 -> Sum3/3
  1/La3/1 -> Sum3/1
  Sum3/1 -> Switch1/3
  mul/1 -> Switch1/1
  mem3/1 -> Log3/2
  Log4/1 -> Switch1/2
  Switch1/1 -> out_2/1
  I6/1 -> Log3/1
  Sum/1 -> mul/2
  mem1/1 -> logic2/1, out_3/1
  Mux/1 -> Fcn/1
  vc/1 -> Relay/1, Sum/1, 1/La3/1, Mux/1
  va/1 -> Sum/2, Sum3/2, Mux/2
  vb/1 -> 1/La4/1, Mux/3
  mul1/1 -> "out_4 "/1
  Fcn/1 -> mul1/2
  logic8/1 -> out_5/1, Log4/1, mem3/1, mul1/1

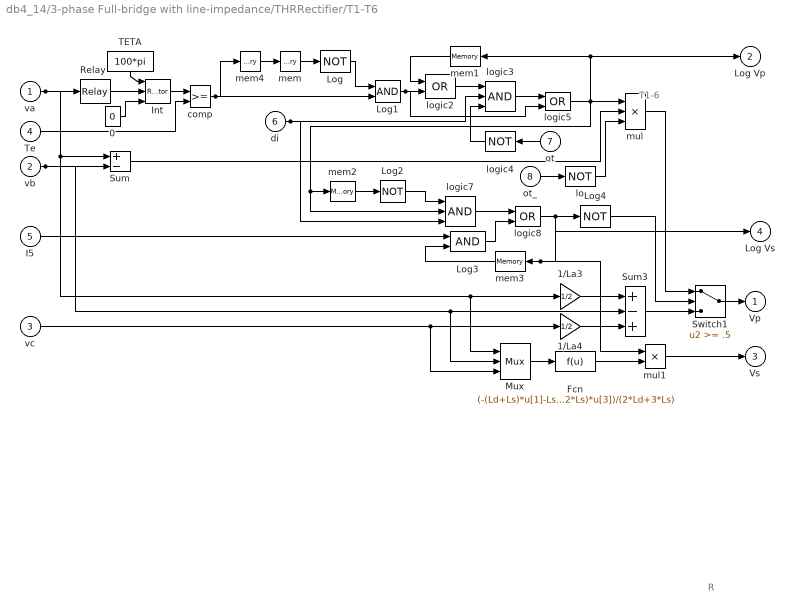
== system db4_14/3-phase Full-bridge with line-impedance/THRRectifier/T1-T6 ==
  note: R
  note: T1-6
  va : Inport
  vb : Inport  Port=2
  vc : Inport  Port=3
  Te : Inport  Port=4
  I5 : Inport  Port=5
  di : Inport  Port=6
  ot : Inport  Port=7
  ot_ : Inport  Port=8
  0 : Constant  Value=0
  1/La3 : Gain  Gain=1/2  SaturateOnIntegerOverflow=on  OutDataTypeStr=Inherit: Same as input  ParamDataTypeStr=Inherit: Same as input
  1/La4 : Gain  Gain=1/2  SaturateOnIntegerOverflow=on  OutDataTypeStr=Inherit: Same as input  ParamDataTypeStr=Inherit: Same as input
  Fcn : Fcn  Expr=(-(Ld+Ls)*u[1]-Ls*u[2]+(Ld+2*Ls)*u[3])/(2*Ld+3*Ls)
  Int : ResetIntegrator
  Log : Logic  Operator=NOT  Inputs=1
  Log1 : Logic
  Log2 : Logic  Operator=NOT  Inputs=1
  Log3 : Logic
  Log4 : Logic  Operator=NOT  Inputs=1
  Mux : Mux  Inputs=3
  Relay : Relay  OnSwitchValue=0  OffSwitchValue=(2^.5)*Vph*sin(pi/6+pi)  OnOutputValue=0  OffOutputValue=1
  Sum : Sum  Inputs=+-  SaturateOnIntegerOverflow=on  InputSameDT=on  OutDataTypeStr=Inherit: Same as first input
  Sum3 : Sum  Inputs=+-+  SaturateOnIntegerOverflow=on  InputSameDT=on  OutDataTypeStr=Inherit: Same as first input
  Switch1 : Switch  Threshold=.5  SaturateOnIntegerOverflow=on  InputSameDT=on
  TETA : Constant  Value=100*pi
  comp : RelationalOperator  RndMeth=Nearest  InputSameDT=on
  lo : Logic  Operator=NOT  Inputs=1
  logic2 : Logic  Operator=OR
  logic3 : Logic  Inputs=3
  logic4 : Logic  Operator=NOT  Inputs=1
  logic5 : Logic  Operator=OR
  logic7 : Logic  Inputs=3
  logic8 : Logic  Operator=OR
  mem{,1..4} (5 alike) : Memory
  mul : Product  Inputs=3  SaturateOnIntegerOverflow=on  RndMeth=Zero  InputSameDT=on  OutDataTypeStr=Inherit: Same as first input
  mul1 : Product  SaturateOnIntegerOverflow=on  RndMeth=Zero  InputSameDT=on  OutDataTypeStr=Inherit: Same as first input
  Vp : Outport
  Log Vp : Outport  Port=2
  Vs : Outport  Port=3
  Log Vs : Outport  Port=4
  wires:
  logic8/1 -> mem3/1, mul1/1, Log4/1, Log Vs/1
  di/1 -> logic7/3, logic3/2
  comp/1 -> Log1/2, mem4/1
  mem4/1 -> mem/1
  lo/1 -> mul/3
  logic4/1 -> logic3/3
  mem1/1 -> logic2/1
  mem/1 -> Log/1
  0/1 -> Int/3
  logic2/1 -> logic3/1
  TETA/1 -> Int/1
  Int/1 -> comp/1
  Te/1 -> comp/2
  ot/1 -> logic4/1
  ot_/1 -> lo/1
  Relay/1 -> Int/2
  logic3/1 -> logic5/1
  Log1/1 -> logic2/2, logic5/2
  logic5/1 -> mul/1, Log Vp/1, mem1/1, mem2/1, logic7/2
  mem2/1 -> Log2/1
  Log/1 -> Log1/1
  Log3/1 -> logic8/2
  logic7/1 -> logic8/1
  Log2/1 -> logic7/1
  1/La4/1 -> Sum3/3
  1/La3/1 -> Sum3/1
  Sum3/1 -> Switch1/3
  mul/1 -> Switch1/1
  mem3/1 -> Log3/2
  Log4/1 -> Switch1/2
  Switch1/1 -> Vp/1
  I5/1 -> Log3/1
  Sum/1 -> mul/2
  Mux/1 -> Fcn/1
  va/1 -> Relay/1, Sum/1, 1/La3/1, Mux/1
  vb/1 -> Sum/2, Sum3/2, Mux/2
  vc/1 -> 1/La4/1, Mux/3
  Fcn/1 -> mul1/2
  mul1/1 -> Vs/1

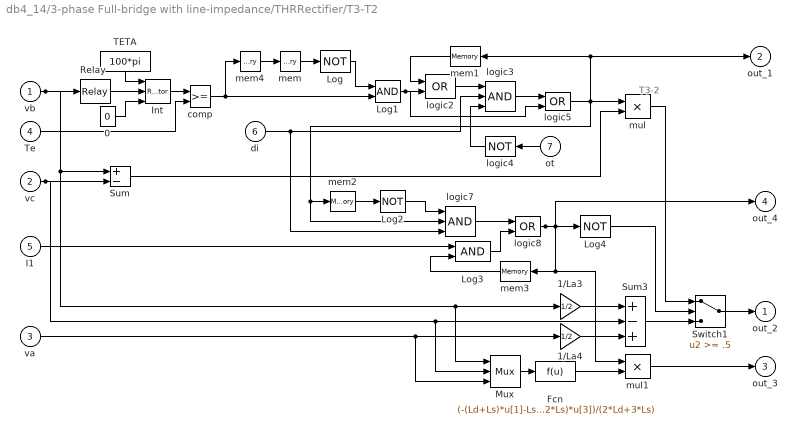
== system db4_14/3-phase Full-bridge with line-impedance/THRRectifier/T3-T2 ==
  note: T3-2
  vb : Inport
  vc : Inport  Port=2
  va : Inport  Port=3
  Te : Inport  Port=4
  I1 : Inport  Port=5
  di : Inport  Port=6
  ot : Inport  Port=7
  0 : Constant  Value=0
  1/La3 : Gain  Gain=1/2  SaturateOnIntegerOverflow=on  OutDataTypeStr=Inherit: Same as input  ParamDataTypeStr=Inherit: Same as input
  1/La4 : Gain  Gain=1/2  SaturateOnIntegerOverflow=on  OutDataTypeStr=Inherit: Same as input  ParamDataTypeStr=Inherit: Same as input
  Fcn : Fcn  Expr=(-(Ld+Ls)*u[1]-Ls*u[2]+(Ld+2*Ls)*u[3])/(2*Ld+3*Ls)
  Int : ResetIntegrator
  Log : Logic  Operator=NOT  Inputs=1
  Log1 : Logic
  Log2 : Logic  Operator=NOT  Inputs=1
  Log3 : Logic
  Log4 : Logic  Operator=NOT  Inputs=1
  Mux : Mux  Inputs=3
  Relay : Relay  OnSwitchValue=0  OffSwitchValue=(2^.5)*Vph*sin(pi/6+pi)  OnOutputValue=0  OffOutputValue=1
  Sum : Sum  Inputs=+-  SaturateOnIntegerOverflow=on  InputSameDT=on  OutDataTypeStr=Inherit: Same as first input
  Sum3 : Sum  Inputs=+-+  SaturateOnIntegerOverflow=on  InputSameDT=on  OutDataTypeStr=Inherit: Same as first input
  Switch1 : Switch  Threshold=.5  SaturateOnIntegerOverflow=on  InputSameDT=on
  TETA : Constant  Value=100*pi
  comp : RelationalOperator  RndMeth=Nearest  InputSameDT=on
  logic2 : Logic  Operator=OR
  logic3 : Logic  Inputs=3
  logic4 : Logic  Operator=NOT  Inputs=1
  logic5 : Logic  Operator=OR
  logic7 : Logic  Inputs=3
  logic8 : Logic  Operator=OR
  mem{,1..4} (5 alike) : Memory
  mul : Product  SaturateOnIntegerOverflow=on  RndMeth=Zero  InputSameDT=on  OutDataTypeStr=Inherit: Same as first input
  mul1 : Product  SaturateOnIntegerOverflow=on  RndMeth=Zero  InputSameDT=on  OutDataTypeStr=Inherit: Same as first input
  out_2 : Outport
  out_1 : Outport  Port=2
  out_3 : Outport  Port=3
  out_4 : Outport  Port=4
  wires:
  comp/1 -> Log1/2, mem4/1
  di/1 -> logic3/2, logic7/3
  mem4/1 -> mem/1
  mem/1 -> Log/1
  Sum/1 -> mul/2
  I1/1 -> Log3/1
  Switch1/1 -> out_2/1
  Log4/1 -> Switch1/2
  logic8/1 -> out_4/1, Log4/1, mem3/1, mul1/1
  mem3/1 -> Log3/2
  mul/1 -> Switch1/1
  Sum3/1 -> Switch1/3
  1/La3/1 -> Sum3/1
  1/La4/1 -> Sum3/3
  logic5/1 -> mul/1, mem2/1, logic7/2, out_1/1, mem1/1
  Log2/1 -> logic7/1
  logic7/1 -> logic8/1
  Log3/1 -> logic8/2
  Log/1 -> Log1/1
  mem2/1 -> Log2/1
  logic3/1 -> logic5/1
  Relay/1 -> Int/2
  ot/1 -> logic4/1
  Te/1 -> comp/2
  Int/1 -> comp/1
  TETA/1 -> Int/1
  logic2/1 -> logic3/1
  0/1 -> Int/3
  Log1/1 -> logic5/2, logic2/2
  mem1/1 -> logic2/1
  logic4/1 -> logic3/3
  Mux/1 -> Fcn/1
  Fcn/1 -> mul1/2
  mul1/1 -> out_3/1
  vb/1 -> Relay/1, Sum/1, 1/La3/1, Mux/1
  vc/1 -> Sum/2, Sum3/2, Mux/2
  va/1 -> 1/La4/1, Mux/3

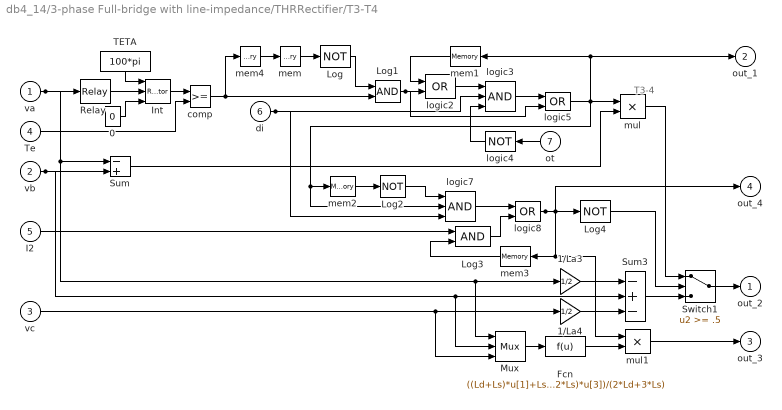
== system db4_14/3-phase Full-bridge with line-impedance/THRRectifier/T3-T4 ==
  note: T3-4
  va : Inport
  vb : Inport  Port=2
  vc : Inport  Port=3
  Te : Inport  Port=4
  I2 : Inport  Port=5
  di : Inport  Port=6
  ot : Inport  Port=7
  0 : Constant  Value=0
  1/La3 : Gain  Gain=1/2  SaturateOnIntegerOverflow=on  OutDataTypeStr=Inherit: Same as input  ParamDataTypeStr=Inherit: Same as input
  1/La4 : Gain  Gain=1/2  SaturateOnIntegerOverflow=on  OutDataTypeStr=Inherit: Same as input  ParamDataTypeStr=Inherit: Same as input
  Fcn : Fcn  Expr=((Ld+Ls)*u[1]+Ls*u[2]-(Ld+2*Ls)*u[3])/(2*Ld+3*Ls)
  Int : ResetIntegrator  InitialCondition=-1
  Log : Logic  Operator=NOT  Inputs=1
  Log1 : Logic
  Log2 : Logic  Operator=NOT  Inputs=1
  Log3 : Logic
  Log4 : Logic  Operator=NOT  Inputs=1
  Mux : Mux  Inputs=3
  Relay : Relay  OnSwitchValue=(2^.5)*Vph*sin(pi/6)  OffSwitchValue=0
  Sum : Sum  Inputs=-+  SaturateOnIntegerOverflow=on  InputSameDT=on  OutDataTypeStr=Inherit: Same as first input
  Sum3 : Sum  Inputs=-+-  SaturateOnIntegerOverflow=on  InputSameDT=on  OutDataTypeStr=Inherit: Same as first input
  Switch1 : Switch  Threshold=.5  SaturateOnIntegerOverflow=on  InputSameDT=on
  TETA : Constant  Value=100*pi
  comp : RelationalOperator  RndMeth=Nearest  InputSameDT=on
  logic2 : Logic  Operator=OR
  logic3 : Logic  Inputs=3
  logic4 : Logic  Operator=NOT  Inputs=1
  logic5 : Logic  Operator=OR
  logic7 : Logic  Inputs=3
  logic8 : Logic  Operator=OR
  mem{,1..4} (5 alike) : Memory
  mul : Product  SaturateOnIntegerOverflow=on  RndMeth=Zero  InputSameDT=on  OutDataTypeStr=Inherit: Same as first input
  mul1 : Product  SaturateOnIntegerOverflow=on  RndMeth=Zero  InputSameDT=on  OutDataTypeStr=Inherit: Same as first input
  out_2 : Outport
  out_1 : Outport  Port=2
  out_3 : Outport  Port=3
  out_4 : Outport  Port=4
  wires:
  comp/1 -> Log1/2, mem4/1
  mem4/1 -> mem/1
  mem/1 -> Log/1
  Sum/1 -> mul/2
  I2/1 -> Log3/1
  Switch1/1 -> out_2/1
  Log4/1 -> Switch1/2
  logic8/1 -> out_4/1, Log4/1, mem3/1, mul1/1
  mem3/1 -> Log3/2
  mul/1 -> Switch1/1
  Sum3/1 -> Switch1/3
  1/La3/1 -> Sum3/1
  1/La4/1 -> Sum3/3
  logic5/1 -> mul/1, mem2/1, logic7/2, out_1/1, mem1/1
  Log2/1 -> logic7/1
  di/1 -> logic3/2, logic7/3
  logic7/1 -> logic8/1
  Log3/1 -> logic8/2
  Log/1 -> Log1/1
  mem2/1 -> Log2/1
  logic3/1 -> logic5/1
  Relay/1 -> Int/2
  ot/1 -> logic4/1
  Te/1 -> comp/2
  Int/1 -> comp/1
  TETA/1 -> Int/1
  logic2/1 -> logic3/1
  0/1 -> Int/3
  Log1/1 -> logic5/2, logic2/2
  mem1/1 -> logic2/1
  logic4/1 -> logic3/3
  Mux/1 -> Fcn/1
  Fcn/1 -> mul1/2
  mul1/1 -> out_3/1
  va/1 -> Relay/1, Sum/1, 1/La3/1, Mux/1
  vb/1 -> Sum/2, Sum3/2, Mux/2
  vc/1 -> 1/La4/1, Mux/3

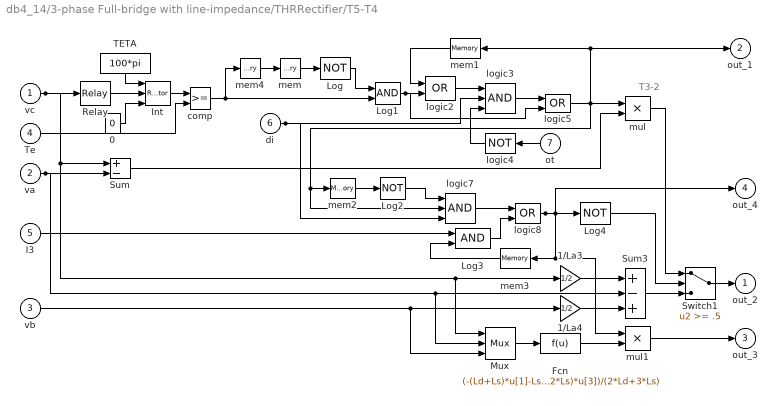
== system db4_14/3-phase Full-bridge with line-impedance/THRRectifier/T5-T4 ==
  note: T3-2
  vc : Inport
  va : Inport  Port=2
  vb : Inport  Port=3
  Te : Inport  Port=4
  I3 : Inport  Port=5
  di : Inport  Port=6
  ot : Inport  Port=7
  0 : Constant  Value=0
  1/La3 : Gain  Gain=1/2  SaturateOnIntegerOverflow=on  OutDataTypeStr=Inherit: Same as input  ParamDataTypeStr=Inherit: Same as input
  1/La4 : Gain  Gain=1/2  SaturateOnIntegerOverflow=on  OutDataTypeStr=Inherit: Same as input  ParamDataTypeStr=Inherit: Same as input
  Fcn : Fcn  Expr=(-(Ld+Ls)*u[1]-Ls*u[2]+(Ld+2*Ls)*u[3])/(2*Ld+3*Ls)
  Int : ResetIntegrator  InitialCondition=2/3*pi
  Log : Logic  Operator=NOT  Inputs=1
  Log1 : Logic
  Log2 : Logic  Operator=NOT  Inputs=1
  Log3 : Logic
  Log4 : Logic  Operator=NOT  Inputs=1
  Mux : Mux  Inputs=3
  Relay : Relay  OnSwitchValue=0  OffSwitchValue=(2^.5)*Vph*sin(pi/6+pi)  OnOutputValue=0  OffOutputValue=1
  Sum : Sum  Inputs=+-  SaturateOnIntegerOverflow=on  InputSameDT=on  OutDataTypeStr=Inherit: Same as first input
  Sum3 : Sum  Inputs=+-+  SaturateOnIntegerOverflow=on  InputSameDT=on  OutDataTypeStr=Inherit: Same as first input
  Switch1 : Switch  Threshold=.5  SaturateOnIntegerOverflow=on  InputSameDT=on
  TETA : Constant  Value=100*pi
  comp : RelationalOperator  RndMeth=Nearest  InputSameDT=on
  logic2 : Logic  Operator=OR
  logic3 : Logic  Inputs=3
  logic4 : Logic  Operator=NOT  Inputs=1
  logic5 : Logic  Operator=OR
  logic7 : Logic  Inputs=3
  logic8 : Logic  Operator=OR
  mem{,1..4} (5 alike) : Memory
  mul : Product  SaturateOnIntegerOverflow=on  RndMeth=Zero  InputSameDT=on  OutDataTypeStr=Inherit: Same as first input
  mul1 : Product  SaturateOnIntegerOverflow=on  RndMeth=Zero  InputSameDT=on  OutDataTypeStr=Inherit: Same as first input
  out_2 : Outport
  out_1 : Outport  Port=2
  out_3 : Outport  Port=3
  out_4 : Outport  Port=4
  wires:
  comp/1 -> Log1/2, mem4/1
  mem4/1 -> mem/1
  mem/1 -> Log/1
  logic4/1 -> logic3/3
  mem1/1 -> logic2/1
  0/1 -> Int/3
  logic2/1 -> logic3/1
  TETA/1 -> Int/1
  Int/1 -> comp/1
  di/1 -> logic7/3, logic3/2
  Te/1 -> comp/2
  ot/1 -> logic4/1
  Relay/1 -> Int/2
  logic3/1 -> logic5/1
  Log1/1 -> logic2/2, logic5/2
  logic5/1 -> mul/1, out_1/1, mem1/1, mem2/1, logic7/2
  mem2/1 -> Log2/1
  Log/1 -> Log1/1
  Log3/1 -> logic8/2
  logic7/1 -> logic8/1
  Log2/1 -> logic7/1
  1/La4/1 -> Sum3/3
  1/La3/1 -> Sum3/1
  Sum3/1 -> Switch1/3
  mul/1 -> Switch1/1
  mem3/1 -> Log3/2
  Log4/1 -> Switch1/2
  Switch1/1 -> out_2/1
  I3/1 -> Log3/1
  Sum/1 -> mul/2
  Mux/1 -> Fcn/1
  vc/1 -> Relay/1, Sum/1, 1/La3/1, Mux/1
  va/1 -> Sum/2, Sum3/2, Mux/2
  vb/1 -> 1/La4/1, Mux/3
  Fcn/1 -> mul1/2
  mul1/1 -> out_3/1
  logic8/1 -> out_4/1, Log4/1, mem3/1, mul1/1

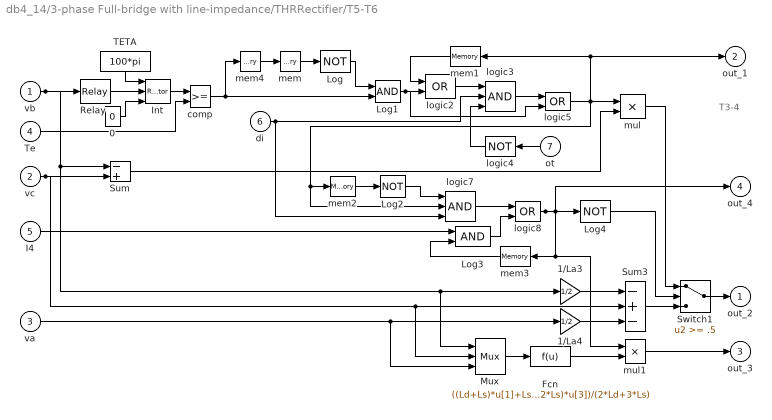
== system db4_14/3-phase Full-bridge with line-impedance/THRRectifier/T5-T6 ==
  note: T3-4
  vb : Inport
  vc : Inport  Port=2
  va : Inport  Port=3
  Te : Inport  Port=4
  I4 : Inport  Port=5
  di : Inport  Port=6
  ot : Inport  Port=7
  0 : Constant  Value=0
  1/La3 : Gain  Gain=1/2  SaturateOnIntegerOverflow=on  OutDataTypeStr=Inherit: Same as input  ParamDataTypeStr=Inherit: Same as input
  1/La4 : Gain  Gain=1/2  SaturateOnIntegerOverflow=on  OutDataTypeStr=Inherit: Same as input  ParamDataTypeStr=Inherit: Same as input
  Fcn : Fcn  Expr=((Ld+Ls)*u[1]+Ls*u[2]-(Ld+2*Ls)*u[3])/(2*Ld+3*Ls)
  Int : ResetIntegrator  InitialCondition=pi/3
  Log : Logic  Operator=NOT  Inputs=1
  Log1 : Logic
  Log2 : Logic  Operator=NOT  Inputs=1
  Log3 : Logic
  Log4 : Logic  Operator=NOT  Inputs=1
  Mux : Mux  Inputs=3
  Relay : Relay  OnSwitchValue=(2^.5)*Vph*sin(pi/6)  OffSwitchValue=0
  Sum : Sum  Inputs=-+  SaturateOnIntegerOverflow=on  InputSameDT=on  OutDataTypeStr=Inherit: Same as first input
  Sum3 : Sum  Inputs=-+-  SaturateOnIntegerOverflow=on  InputSameDT=on  OutDataTypeStr=Inherit: Same as first input
  Switch1 : Switch  Threshold=.5  SaturateOnIntegerOverflow=on  InputSameDT=on
  TETA : Constant  Value=100*pi
  comp : RelationalOperator  RndMeth=Nearest  InputSameDT=on
  logic2 : Logic  Operator=OR
  logic3 : Logic  Inputs=3
  logic4 : Logic  Operator=NOT  Inputs=1
  logic5 : Logic  Operator=OR
  logic7 : Logic  Inputs=3
  logic8 : Logic  Operator=OR
  mem{,1..4} (5 alike) : Memory
  mul : Product  SaturateOnIntegerOverflow=on  RndMeth=Zero  InputSameDT=on  OutDataTypeStr=Inherit: Same as first input
  mul1 : Product  SaturateOnIntegerOverflow=on  RndMeth=Zero  InputSameDT=on  OutDataTypeStr=Inherit: Same as first input
  out_2 : Outport
  out_1 : Outport  Port=2
  out_3 : Outport  Port=3
  out_4 : Outport  Port=4
  wires:
  comp/1 -> Log1/2, mem4/1
  mem4/1 -> mem/1
  mem/1 -> Log/1
  Sum/1 -> mul/2
  I4/1 -> Log3/1
  Switch1/1 -> out_2/1
  Log4/1 -> Switch1/2
  logic8/1 -> out_4/1, Log4/1, mem3/1, mul1/1
  mem3/1 -> Log3/2
  mul/1 -> Switch1/1
  Sum3/1 -> Switch1/3
  1/La3/1 -> Sum3/1
  1/La4/1 -> Sum3/3
  logic5/1 -> mul/1, mem2/1, logic7/2, out_1/1, mem1/1
  Log2/1 -> logic7/1
  di/1 -> logic3/2, logic7/3
  logic7/1 -> logic8/1
  Log3/1 -> logic8/2
  Log/1 -> Log1/1
  mem2/1 -> Log2/1
  logic3/1 -> logic5/1
  Relay/1 -> Int/2
  ot/1 -> logic4/1
  Te/1 -> comp/2
  Int/1 -> comp/1
  TETA/1 -> Int/1
  logic2/1 -> logic3/1
  0/1 -> Int/3
  Log1/1 -> logic5/2, logic2/2
  mem1/1 -> logic2/1
  logic4/1 -> logic3/3
  Mux/1 -> Fcn/1
  Fcn/1 -> mul1/2
  mul1/1 -> out_3/1
  vb/1 -> Relay/1, Sum/1, 1/La3/1, Mux/1
  vc/1 -> Sum/2, Sum3/2, Mux/2
  va/1 -> 1/La4/1, Mux/3

== system db4_14/Cascade Control for PMDCM Controlled Rectifier 4 quadrants /Conmutator/Cont ==
  in_2 : Inport
  Constant : Constant  Value=0
  Constant1 : Constant
  Constant2 : Constant  Value=.01
  Logical Operator1 : Logic  Operator=NOT  Inputs=1
  Logical Operator12 : Logic  Operator=OR
  Logical Operator2 : Logic  Operator=NOT  Inputs=1
  Logical Operator3 : Logic
  Memory : Memory  InitialCondition=1
  Product : Product  SaturateOnIntegerOverflow=on  RndMeth=Zero  InputSameDT=on  OutDataTypeStr=Inherit: Same as first input
  Product1 : Product  SaturateOnIntegerOverflow=on  RndMeth=Zero  InputSameDT=on  OutDataTypeStr=Inherit: Same as first input
  Relational Operator : RelationalOperator  Operator=<=  RndMeth=Nearest  InputSameDT=on
  Reset Integrator : ResetIntegrator  InitialCondition=.0099
  out_1 : Outport
  wires:
  Constant2/1 -> Relational Operator/1
  Relational Operator/1 -> out_1/1, Logical Operator2/1
  in_2/1 -> Logical Operator12/1
  Constant1/1 -> Product/1
  Product/1 -> Reset Integrator/1
  Logical Operator1/1 -> Reset Integrator/2
  Constant/1 -> Reset Integrator/3
  Product1/1 -> Relational Operator/2
  Logical Operator12/1 -> Logical Operator1/1, Product1/2, Logical Operator3/1, Product/2
  Memory/1 -> Logical Operator12/2
  Logical Operator3/1 -> Memory/1
  Logical Operator2/1 -> Logical Operator3/2
  Reset Integrator/1 -> Product1/1

== system db4_14/Cascade Control for PMDCM Controlled Rectifier 4 quadrants /Conmutator/Paso por Cero ==
  Ir : Inport
  Cont : Inport  Port=2
  Constant : Constant  Value=0
  Logical Operator{1,4..6} (4 alike) : Logic
  Logical Operator2 : Logic  Operator=OR
  Logical Operator3 : Logic  Operator=OR  Inputs=3
  Logical Operator7 : Logic  Operator=NOT  Inputs=1
  Memory : Memory
  Memory2 : Memory  InitialCondition=1
  Relational Operator : RelationalOperator  Operator=>  RndMeth=Nearest  InputSameDT=on
  Relational Operator1 : RelationalOperator  Operator=<  RndMeth=Nearest  InputSameDT=on
  Relational Operator2 : RelationalOperator  Operator=~=  RndMeth=Nearest  InputSameDT=on
  Relational Operator3 : RelationalOperator  Operator===  RndMeth=Nearest  InputSameDT=on
  Relational Operator4 : RelationalOperator  Operator=>  RndMeth=Nearest  InputSameDT=on
  Relational Operator5 : RelationalOperator  Operator=<  RndMeth=Nearest  InputSameDT=on
  Ir = 0 : Outport
  wires:
  Memory2/1 -> Ir = 0/1, Logical Operator1/1
  Logical Operator2/1 -> Memory2/1
  Logical Operator1/1 -> Logical Operator2/2
  Logical Operator7/1 -> Logical Operator1/2
  Cont/1 -> Logical Operator7/1
  Logical Operator4/1 -> Logical Operator3/3
  Logical Operator6/1 -> Logical Operator3/1
  Logical Operator5/1 -> Logical Operator3/2
  Relational Operator5/1 -> Logical Operator6/1
  Relational Operator4/1 -> Logical Operator6/2
  Memory/1 -> Relational Operator4/1, Relational Operator1/1, Relational Operator2/2
  Relational Operator1/1 -> Logical Operator5/2
  Relational Operator/1 -> Logical Operator5/1
  Relational Operator3/1 -> Logical Operator4/2
  Relational Operator2/1 -> Logical Operator4/1
  Ir/1 -> Relational Operator3/2, Memory/1, Relational Operator5/1, Relational Operator/1
  Constant/1 -> Relational Operator4/2, Relational Operator5/2, Relational Operator1/2, Relational Operator3/1, Relational Operator2/1, Relational Operator/2
  Logical Operator3/1 -> Logical Operator2/1

== system db4_14/Cascade Control for PMDCM Controlled Rectifier 4 quadrants /i - Controller/I -ctrl ==
  in_2 : Inport
  in_1 : Inport  Port=2
  3 : Constant  Value=0
  Gain : Gain  Gain=Kpi/TIi  SaturateOnIntegerOverflow=on  OutDataTypeStr=Inherit: Same as input  ParamDataTypeStr=Inherit: Same as input
  Gain1 : Gain  Gain=Kpi  SaturateOnIntegerOverflow=on  OutDataTypeStr=Inherit: Same as input  ParamDataTypeStr=Inherit: Same as input
  Gain2 : Gain  Gain=100*Kpi/TIi  SaturateOnIntegerOverflow=on  OutDataTypeStr=Inherit: Same as input  ParamDataTypeStr=Inherit: Same as input
  Limited Integrator : Integrator  LimitOutput=on  UpperSaturationLimit=514.598  LowerSaturationLimit=-514.598
  Sum : Sum  SaturateOnIntegerOverflow=on  InputSameDT=on  OutDataTypeStr=Inherit: Same as first input
  Switch : Switch  Threshold=.5  SaturateOnIntegerOverflow=on  InputSameDT=on
  Switch1 : Switch  Threshold=.5  SaturateOnIntegerOverflow=on  InputSameDT=on
  out_1 : Outport
  wires:
  Switch1/1 -> Sum/2
  Limited Integrator/1 -> Sum/1
  in_2/1 -> Switch1/2, Switch/2
  3/1 -> Switch1/3
  Gain1/1 -> Switch1/1
  Gain2/1 -> Switch/3
  Switch/1 -> Limited Integrator/1
  Gain/1 -> Switch/1
  in_1/1 -> Gain2/1, Gain/1, Gain1/1
  Sum/1 -> out_1/1

== system db4_14/Permanent Magnet PMDCM/Converter with Zs 2 & 4 Quadrants/Subsystem ==
  In1 : Inport
  In2 : Inport  Port=2
  Gain1 : Gain  Gain=-1  SaturateOnIntegerOverflow=on  OutDataTypeStr=Inherit: Same as input  ParamDataTypeStr=Inherit: Same as input
  Switch3 : Switch  Threshold=.5  SaturateOnIntegerOverflow=on  InputSameDT=on
  Out1 : Outport
  wires:
  In2/1 -> Switch3/2
  Switch3/1 -> Out1/1
  In1/1 -> Gain1/1, Switch3/1
  Gain1/1 -> Switch3/3
